simulink model "fuzzycontrol_sim"  (R2017a)
settings: Solver=FixedStepAuto  StartTime=0.0  StopTime=200  FixedStep=0.1  RelTol=1e-3
undefined symbols (not defined in the file): Humusoft, MF644, T_f, Ts
libraries: sldrtlib x5, fuzblock x1
settings Model: Creator=CSE2017  LastModifiedBy=CSE2017

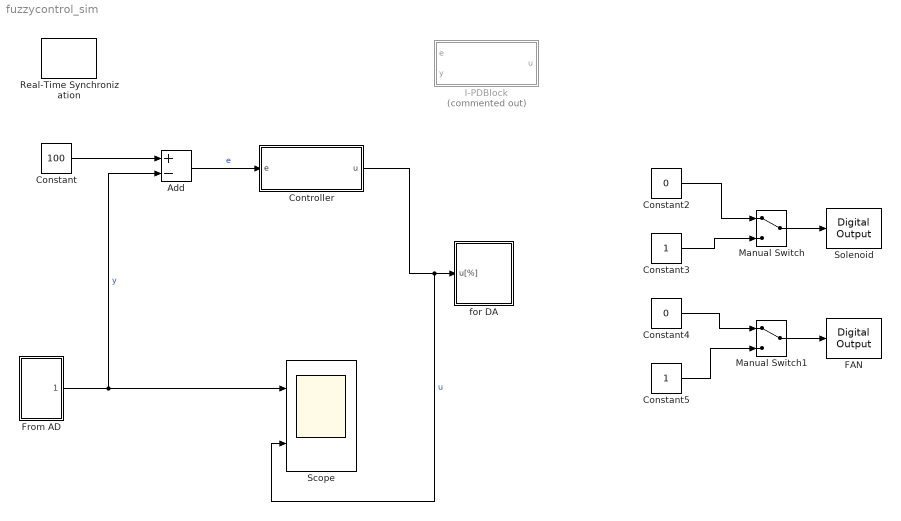
== system fuzzycontrol_sim ==
  Add : Sum  Inputs=+-
  Constant : Constant  Value=100
  Constant2 : Constant  Value=0
  Constant3 : Constant
  Constant4 : Constant  Value=0
  Constant5 : Constant
  Controller : Subsystem
  FAN : sldrtlib/Digital Output  SampleTime=Ts  MaxMissedTicks=10  ShowMissedTicks=off  YieldWhenWaiting=off  DrvName=Humusoft/MF644  DrvAddress=4294967295  DrvOptions=0  Channels=2  BitMode=1  InitialValue=0  FinalValue=1
      settings: AttributesFormatString=Humusoft\nMF644 [auto]  SourceProductName=Simulink Desktop Real-Time  SourceProductBaseCode=WT
  From AD : Subsystem
  I-PDBlock : Subsystem  Commented=on
  Manual Switch : ManualSwitch
  Manual Switch1 : ManualSwitch
  Real-Time Synchronization : sldrtlib/Real-Time Synchronization  SampleTime=Ts  MaxMissedTicks=10  ShowMissedTicks=off  YieldWhenWaiting=off
  Scope : Scope  NumInputPorts=2
  Solenoid : sldrtlib/Digital Output  SampleTime=Ts  MaxMissedTicks=10  ShowMissedTicks=off  YieldWhenWaiting=off  DrvName=Humusoft/MF644  DrvAddress=4294967295  DrvOptions=0  Channels=1  BitMode=1  InitialValue=0  FinalValue=0
      settings: AttributesFormatString=Humusoft\nMF644 [auto]  SourceProductName=Simulink Desktop Real-Time  SourceProductBaseCode=WT
  for DA : Subsystem
  wires:
  Constant2/1 -> Manual Switch/1
  Constant3/1 -> Manual Switch/2
  Constant4/1 -> Manual Switch1/1
  Constant5/1 -> Manual Switch1/2
  Manual Switch1/1 -> FAN/1
  Manual Switch/1 -> Solenoid/1
  From AD/1(y[deg.]) -> Add/2, Scope/1  "y"
  Constant/1 -> Add/1
  Add/1 -> Controller/1("e ")  "e"
  Controller/1(u) -> Scope/2, for DA/1(u[%])  "u"

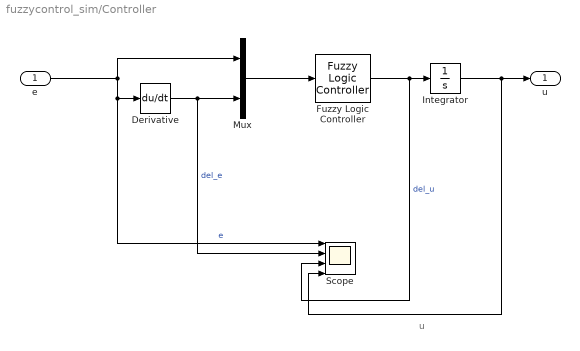
== system fuzzycontrol_sim/Controller ==
  note: u
  "e " : Inport
  Derivative : Derivative
  Fuzzy Logic Controller : fuzblock/Fuzzy Logic  Controller  fis=ff
  Integrator : Integrator  InitialCondition=30  LimitOutput=on  UpperSaturationLimit=30  LowerSaturationLimit=0
  Mux : Mux  Inputs=2
  Scope : Scope  NumInputPorts=4
  u : Outport
  wires:
  "e "/1 -> Mux/1, Derivative/1, Scope/1  "e"
  Mux/1 -> Fuzzy Logic Controller/1
  Fuzzy Logic Controller/1 -> Scope/3, Integrator/1  "del_u"
  Integrator/1 -> Scope/4, u/1
  Derivative/1 -> Scope/2, Mux/2  "del_e"

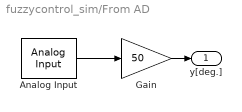
== system fuzzycontrol_sim/From AD ==
  Analog Input : sldrtlib/Analog Input  SampleTime=0.1  MaxMissedTicks=10  ShowMissedTicks=off  YieldWhenWaiting=off  DrvName=Humusoft/MF644  DrvAddress=4294967295  DrvOptions=0  Channels=1  RangeMode=1  VoltRange=1  DataType=1
      settings: AttributesFormatString=Humusoft\nMF644 [auto]  SourceProductName=Simulink Desktop Real-Time
  Gain : Gain  Gain=50
  y[deg.] : Outport
  wires:
  Gain/1 -> y[deg.]/1
  Analog Input/1 -> Gain/1

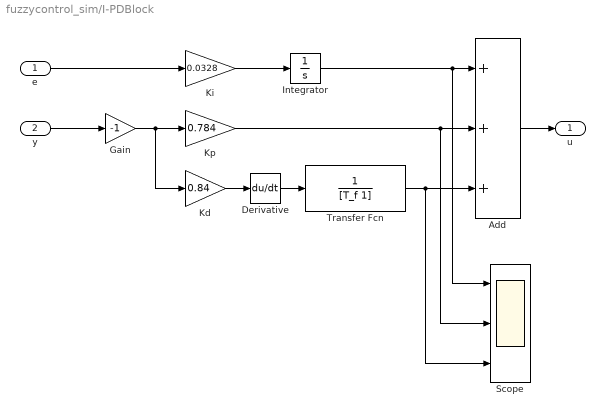
== system fuzzycontrol_sim/I-PDBlock ==
  e : Inport
  "y " : Inport  Port=2
  Add : Sum  Inputs=+++
  Derivative : Derivative
  Gain : Gain  Gain=-1
  Integrator : Integrator
  Kd : Gain  Gain=0.84
  Ki : Gain  Gain=0.0328
  "Kp " : Gain  Gain=0.784
  Scope : Scope  NumInputPorts=3
  Transfer Fcn : TransferFcn  Denominator=[T_f 1]
  u : Outport
  wires:
  Kd/1 -> Derivative/1
  Ki/1 -> Integrator/1
  "Kp "/1 -> Scope/2, Add/2
  Derivative/1 -> Transfer Fcn/1
  e/1 -> Ki/1
  Add/1 -> u/1
  "y "/1 -> Gain/1
  Gain/1 -> Kd/1, "Kp "/1
  Integrator/1 -> Scope/1, Add/1
  Transfer Fcn/1 -> Scope/3, Add/3

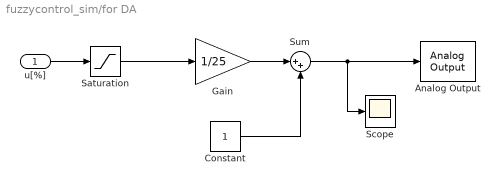
== system fuzzycontrol_sim/for DA ==
  u[%] : Inport
  "Analog Output " : sldrtlib/Analog Output  SampleTime=0.1  MaxMissedTicks=10  ShowMissedTicks=off  YieldWhenWaiting=off  DrvName=Humusoft/MF644  DrvAddress=4294967295  DrvOptions=0  Channels=1  RangeMode=1  VoltRange=1  InitialValue=1  FinalValue=1
      settings: AttributesFormatString=Humusoft\nMF644 [auto]  SourceProductName=Simulink Desktop Real-Time
  Constant : Constant
  Gain : Gain  Gain=1/25
  Saturation : Saturate  UpperLimit=100  LowerLimit=0
  Scope : Scope
  Sum : Sum  Inputs=|++
  wires:
  Gain/1 -> Sum/1
  Sum/1 -> Scope/1, "Analog Output "/1
  Constant/1 -> Sum/2
  u[%]/1 -> Saturation/1
  Saturation/1 -> Gain/1
